simulink model "TOGGLER"  (R2022b)
settings: Solver=FixedStepDiscrete  StartTime=0  StopTime=duration  FixedStep=sample_time  RelTol=1e-3
values from neighbouring files (symbols this model uses):
  CTRL =     [TOGGLER_params.mat]
  CTRLSector =     [TOGGLER_params.mat]
  Greedy_Status = 1    [TOGGLER_params.mat]    (also in init_TOGGLER.m = logical(true))
  sample_time = 0.1    [TOGGLER_params.mat]
  WFC_1_Status = 1    [TOGGLER_params.mat]    (also in init_TOGGLER.m = logical(true))
  WFC_2_Status = 1    [TOGGLER_params.mat]    (also in init_TOGGLER.m = logical(true))
  WFC_3_Status = 1    [TOGGLER_params.mat]    (also in init_TOGGLER.m = logical(true))
undefined symbols (not defined in the file or in its folder): j
libraries: simulink x39, dspindex x14, dspstat3 x4, dspsigops x1
(part 2 of 2)

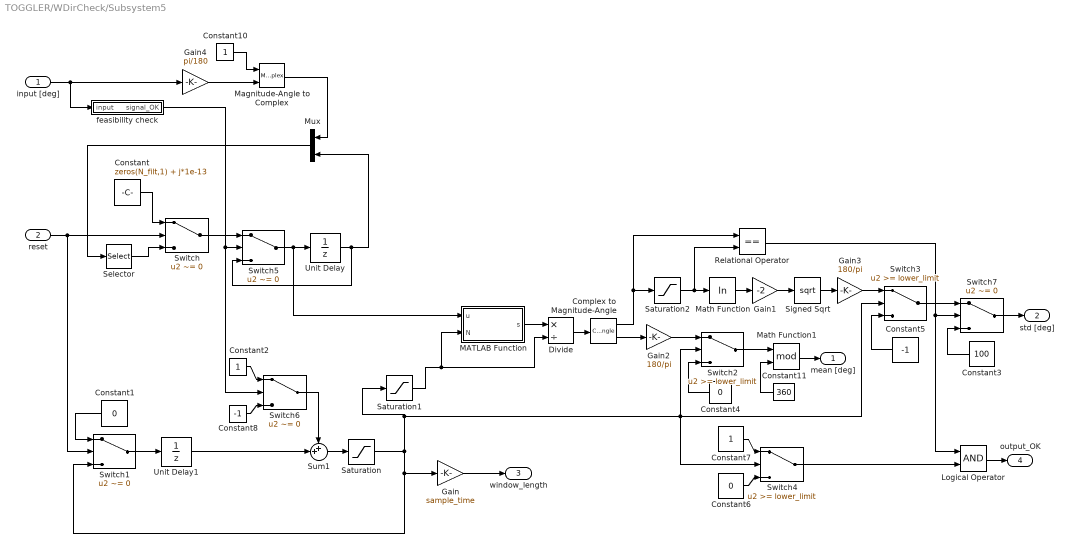
== system TOGGLER/WDirCheck/Subsystem5 ==
  input [deg] : Inport
  reset : Inport  Port=2
  Complex to Magnitude-Angle : ComplexToMagnitudeAngle
  Constant : Constant  Value=zeros(N_filt,1) + j*1e-13  SampleTime=sample_time
  Constant1 : Constant  Value=0  SampleTime=sample_time
  Constant10 : Constant  SampleTime=sample_time
  Constant11 : Constant  Value=360
  Constant2 : Constant  SampleTime=sample_time
  Constant3 : Constant  Value=100  SampleTime=sample_time
  Constant4 : Constant  Value=0  SampleTime=sample_time
  Constant5 : Constant  Value=-1  SampleTime=sample_time
  Constant6 : Constant  Value=0  OutDataTypeStr=boolean  SampleTime=sample_time
  Constant7 : Constant  OutDataTypeStr=boolean  SampleTime=sample_time
  Constant8 : Constant  Value=-1  SampleTime=sample_time
  Divide : Product  Inputs=*/
  Gain : Gain  Gain=sample_time
  Gain1 : Gain  Gain=-2
  Gain2 : Gain  Gain=180/pi
  Gain3 : Gain  Gain=180/pi
  Gain4 : Gain  Gain=pi/180
  Logical Operator : Logic  AllPortsSameDT=off  OutDataTypeStr=boolean
  MATLAB Function : MATLAB Function  TreatAsAtomicUnit=on
  Magnitude-Angle to Complex : MagnitudeAngleToComplex
  Math Function : Math  Operator=log  SignedPower=on
  Math Function1 : Math  Operator=mod  SignedPower=on
  Mux : Mux  Inputs=2
  Relational Operator : RelationalOperator  Operator===  OutDataTypeStr=boolean  RndMeth=Simplest  InputSameDT=off
  Saturation : Saturate  UpperLimit=N_filt  LowerLimit=0
  Saturation1 : Saturate  UpperLimit=N_filt  LowerLimit=lower_limit
  Saturation2 : Saturate  UpperLimit=1  LowerLimit=1e-7
  Selector : Selector  InputPortWidth=N_filt+1  IndexOptions=Index vector (dialog)  Indices=1:N_filt  OutputSizes=1
  Signed Sqrt : Sqrt
  Sum1 : Sum  Inputs=++|
  Switch{,1,5..6} (4 alike) : Switch  Criteria=u2 ~= 0  SaturateOnIntegerOverflow=off  InputSameDT=off
  Switch2 : Switch  Threshold=lower_limit  SaturateOnIntegerOverflow=off  InputSameDT=off
  Switch3 : Switch  Threshold=lower_limit  SaturateOnIntegerOverflow=off  InputSameDT=off
  Switch4 : Switch  Threshold=lower_limit  SaturateOnIntegerOverflow=off  InputSameDT=off
  Switch7 : Switch  Criteria=u2 ~= 0  Threshold=lower_limit  SaturateOnIntegerOverflow=off  InputSameDT=off
  Unit Delay : UnitDelay  InitialCondition=zeros(N_filt,1)  SampleTime=sample_time  HasFrameUpgradeWarning=on
  Unit Delay1 : UnitDelay  SampleTime=sample_time  HasFrameUpgradeWarning=on
  feasibility check : Subsystem
  mean [deg] : Outport
  std [deg] : Outport  Port=2
  window_length : Outport  Port=3
  output_OK : Outport  Port=4
  wires:
  Math Function1/1 -> mean [deg]/1
  Switch2/1 -> Math Function1/1
  Constant11/1 -> Math Function1/2
  Saturation2/1 -> Math Function/1, Relational Operator/2
  Gain3/1 -> Switch3/1
  Gain4/1 -> Magnitude-Angle to Complex/2
  input [deg]/1 -> Gain4/1, feasibility check/1(input)
  Gain2/1 -> Switch2/1
  Switch5/1 -> Unit Delay/1, MATLAB Function/1(u)
  Switch6/1 -> Sum1/1
  Constant7/1 -> Switch4/1
  Constant6/1 -> Switch4/3
  Constant1/1 -> Switch1/1
  Constant/1 -> Switch/1
  Selector/1 -> Switch/3
  Gain/1 -> window_length/1
  MATLAB Function/1(s) -> Divide/1
  Sum1/1 -> Saturation/1
  Signed Sqrt/1 -> Gain3/1
  Constant5/1 -> Switch3/3
  Switch1/1 -> Unit Delay1/1
  Switch3/1 -> Switch7/1
  Constant4/1 -> Switch2/3
  Unit Delay/1 -> Switch5/3, Mux/2
  Mux/1 -> Selector/1
  Saturation1/1 -> Divide/2, MATLAB Function/2(N)
  reset/1 -> Switch/2, Switch1/2
  Unit Delay1/1 -> Sum1/2
  Saturation/1 -> Gain/1, Switch1/3, Switch2/2, Switch4/2, Switch3/2, Saturation1/1
  feasibility check/1(signal_OK) -> Switch6/2, Switch5/2
  Switch/1 -> Switch5/1
  Constant2/1 -> Switch6/1
  Constant8/1 -> Switch6/3
  Magnitude-Angle to Complex/1 -> Mux/1
  Constant10/1 -> Magnitude-Angle to Complex/1
  Divide/1 -> Complex to Magnitude-Angle/1
  Complex to Magnitude-Angle/2 -> Gain2/1
  Complex to Magnitude-Angle/1 -> Saturation2/1, Relational Operator/1
  Math Function/1 -> Gain1/1
  Gain1/1 -> Signed Sqrt/1
  Logical Operator/1 -> output_OK/1
  Switch4/1 -> Logical Operator/2
  Relational Operator/1 -> Switch7/2, Logical Operator/1
  Constant3/1 -> Switch7/3
  Switch7/1 -> std [deg]/1

== system TOGGLER/Check Input/Subsystem5/Subsystem5 ==
  In1 : Inport
  Abs : Abs  SaturateOnIntegerOverflow=off
  Compare To Constant : simulink/Logic and Bit Operations/Compare To Constant  relop=<=  const=0.00001  OutDataTypeStr=boolean
  IsInf : RelationalOperator  Operator=isInf  OutDataTypeStr=boolean  RndMeth=Simplest  InputSameDT=off
  IsNaN : RelationalOperator  Operator=isNaN  OutDataTypeStr=boolean  RndMeth=Simplest  InputSameDT=off
  Logical Operator : Logic  Operator=OR  Inputs=3  AllPortsSameDT=off  OutDataTypeStr=boolean
  ErrorFlag : Outport  VectorParamsAs1DForOutWhenUnconnected=off
  wires:
  Abs/1 -> Compare To Constant/1
  Compare To Constant/1 -> Logical Operator/1
  Logical Operator/1 -> ErrorFlag/1
  IsInf/1 -> Logical Operator/3
  In1/1 -> IsInf/1, IsNaN/1, Abs/1
  IsNaN/1 -> Logical Operator/2

== system TOGGLER/Check Input/Subsystem6/Subsystem5 ==
  In1 : Inport
  Abs : Abs  SaturateOnIntegerOverflow=off
  Compare To Constant : simulink/Logic and Bit Operations/Compare To Constant  relop=<=  const=0.00001  OutDataTypeStr=boolean
  IsInf : RelationalOperator  Operator=isInf  OutDataTypeStr=boolean  RndMeth=Simplest  InputSameDT=off
  IsNaN : RelationalOperator  Operator=isNaN  OutDataTypeStr=boolean  RndMeth=Simplest  InputSameDT=off
  Logical Operator : Logic  Operator=OR  Inputs=3  AllPortsSameDT=off  OutDataTypeStr=boolean
  ErrorFlag : Outport  VectorParamsAs1DForOutWhenUnconnected=off
  wires:
  IsNaN/1 -> Logical Operator/2
  In1/1 -> Abs/1, IsNaN/1, IsInf/1
  IsInf/1 -> Logical Operator/3
  Logical Operator/1 -> ErrorFlag/1
  Compare To Constant/1 -> Logical Operator/1
  Abs/1 -> Compare To Constant/1

== system TOGGLER/CheckSectorsInflow/Atomic Subsystem/CheckRangeMisal ==
  VariableToCheck : Inport
  VarRange : Inport  Port=2  OutDataTypeStr=double
  IdxToCheck : Inport  Port=3
  Interval Test Dynamic : simulink/Logic and Bit Operations/Interval Test Dynamic  IntervalClosedRight=on  IntervalClosedLeft=on  OutDataTypeStr=boolean
  Scope : Scope  NumInputPorts=2
  Variable Selector3 : dspindex/Variable Selector  NumInputs=1  rowsOrCols=Rows  IdxMode=Variable  Elements=[1 3]  ZerOneIdxMode=One-based  errmode=Clip Index  FillMode=on  FillValues=0
  Zero : Constant  Value=0  OutDataTypeStr=Inherit: Inherit via back propagation
  Flag_InRange : Outport  VectorParamsAs1DForOutWhenUnconnected=off
  wires:
  IdxToCheck/1 -> Variable Selector3/2
  Interval Test Dynamic/1 -> Scope/1, Flag_InRange/1
  VarRange/1 -> Variable Selector3/1
  Variable Selector3/1 -> Interval Test Dynamic/1
  VariableToCheck/1 -> Scope/2, Interval Test Dynamic/2
  Zero/1 -> Interval Test Dynamic/3

== system TOGGLER/CheckSectorsInflow/Atomic Subsystem/CheckRangeNacelle ==
  VariableToCheck : Inport
  VarRange : Inport  Port=2  OutDataTypeStr=double
  IdxToCheck : Inport  Port=3
  Multiport Selector : dspindex/Multiport Selector  rowsOrCols=Columns  idxCellArray={ 1,2}  idxErrMode=Clip Index
  Scope : Scope  NumInputPorts=2
  Subsystem : Subsystem
  Variable Selector3 : dspindex/Variable Selector  NumInputs=1  rowsOrCols=Rows  IdxMode=Variable  Elements=[1 3]  ZerOneIdxMode=One-based  errmode=Clip Index  FillMode=on  FillValues=0
  Flag_InRange : Outport  VectorParamsAs1DForOutWhenUnconnected=off
  wires:
  IdxToCheck/1 -> Variable Selector3/2
  Multiport Selector/1 -> Subsystem/3(LowerBound)
  Subsystem/1(AngleInRange) -> Scope/1, Flag_InRange/1
  VarRange/1 -> Variable Selector3/1
  Variable Selector3/1 -> Multiport Selector/1
  Multiport Selector/2 -> Subsystem/1(UpperBound)
  VariableToCheck/1 -> Subsystem/2(Angle), Scope/2

== system TOGGLER/CheckSectorsInflow/Atomic Subsystem/CheckRangeWDir ==
  VariableToCheck : Inport
  VarRange : Inport  Port=2  OutDataTypeStr=double
  IdxToCheck : Inport  Port=3
  Multiport Selector : dspindex/Multiport Selector  rowsOrCols=Columns  idxCellArray={ 1,2}  idxErrMode=Clip Index
  Scope : Scope
  Subsystem : Subsystem
  Variable Selector3 : dspindex/Variable Selector  NumInputs=1  rowsOrCols=Rows  IdxMode=Variable  Elements=[1 3]  ZerOneIdxMode=One-based  errmode=Clip Index  FillMode=on  FillValues=0
  Flag_InRange : Outport  VectorParamsAs1DForOutWhenUnconnected=off
  wires:
  IdxToCheck/1 -> Variable Selector3/2
  Multiport Selector/1 -> Subsystem/3(LowerBound)
  VarRange/1 -> Variable Selector3/1
  Variable Selector3/1 -> Multiport Selector/1
  Multiport Selector/2 -> Subsystem/1(UpperBound)
  VariableToCheck/1 -> Subsystem/2(Angle)
  Subsystem/1(AngleInRange) -> Scope/1, Flag_InRange/1

== system TOGGLER/CheckSectorsInflow/Atomic Subsystem/CheckRangeWS ==
  VariableToCheck : Inport
  VarRange : Inport  Port=2  OutDataTypeStr=double
  IdxToCheck : Inport  Port=3
  Interval Test Dynamic : simulink/Logic and Bit Operations/Interval Test Dynamic  IntervalClosedRight=on  IntervalClosedLeft=on  OutDataTypeStr=boolean
  Multiport Selector : dspindex/Multiport Selector  rowsOrCols=Columns  idxCellArray={ 1,2}  idxErrMode=Clip Index
  Scope : Scope  NumInputPorts=2
  Variable Selector3 : dspindex/Variable Selector  NumInputs=1  rowsOrCols=Rows  IdxMode=Variable  Elements=[1 3]  ZerOneIdxMode=One-based  errmode=Clip Index  FillMode=on  FillValues=0
  Flag_InRange : Outport  VectorParamsAs1DForOutWhenUnconnected=off
  wires:
  IdxToCheck/1 -> Variable Selector3/2
  Multiport Selector/1 -> Interval Test Dynamic/3
  Interval Test Dynamic/1 -> Scope/2, Flag_InRange/1
  VarRange/1 -> Scope/1, Variable Selector3/1
  Variable Selector3/1 -> Multiport Selector/1
  Multiport Selector/2 -> Interval Test Dynamic/1
  VariableToCheck/1 -> Interval Test Dynamic/2

== system TOGGLER/CheckSectorsInflow/Atomic Subsystem1/CheckRangeMisal ==
  VariableToCheck : Inport
  VarRange : Inport  Port=2  OutDataTypeStr=double
  IdxToCheck : Inport  Port=3
  Interval Test Dynamic : simulink/Logic and Bit Operations/Interval Test Dynamic  IntervalClosedRight=on  IntervalClosedLeft=on  OutDataTypeStr=boolean
  Scope : Scope  NumInputPorts=2
  Variable Selector3 : dspindex/Variable Selector  NumInputs=1  rowsOrCols=Rows  IdxMode=Variable  Elements=[1 3]  ZerOneIdxMode=One-based  errmode=Clip Index  FillMode=on  FillValues=0
  Zero : Constant  Value=0  OutDataTypeStr=Inherit: Inherit via back propagation
  Flag_InRange : Outport  VectorParamsAs1DForOutWhenUnconnected=off
  wires:
  Zero/1 -> Interval Test Dynamic/3
  VariableToCheck/1 -> Interval Test Dynamic/2, Scope/2
  Variable Selector3/1 -> Interval Test Dynamic/1
  VarRange/1 -> Variable Selector3/1
  Interval Test Dynamic/1 -> Flag_InRange/1, Scope/1
  IdxToCheck/1 -> Variable Selector3/2

== system TOGGLER/CheckSectorsInflow/Atomic Subsystem1/CheckRangeNacelle ==
  VariableToCheck : Inport
  VarRange : Inport  Port=2  OutDataTypeStr=double
  IdxToCheck : Inport  Port=3
  Multiport Selector : dspindex/Multiport Selector  rowsOrCols=Columns  idxCellArray={ 1,2}  idxErrMode=Clip Index
  Scope : Scope  NumInputPorts=2
  Subsystem : Subsystem
  Variable Selector3 : dspindex/Variable Selector  NumInputs=1  rowsOrCols=Rows  IdxMode=Variable  Elements=[1 3]  ZerOneIdxMode=One-based  errmode=Clip Index  FillMode=on  FillValues=0
  Flag_InRange : Outport  VectorParamsAs1DForOutWhenUnconnected=off
  wires:
  VariableToCheck/1 -> Subsystem/2(Angle), Scope/2
  Variable Selector3/1 -> Multiport Selector/1
  VarRange/1 -> Variable Selector3/1
  Subsystem/1(AngleInRange) -> Scope/1, Flag_InRange/1
  IdxToCheck/1 -> Variable Selector3/2
  Multiport Selector/1 -> Subsystem/3(LowerBound)
  Multiport Selector/2 -> Subsystem/1(UpperBound)

== system TOGGLER/CheckSectorsInflow/Atomic Subsystem1/CheckRangeWDir ==
  VariableToCheck : Inport
  VarRange : Inport  Port=2  OutDataTypeStr=double
  IdxToCheck : Inport  Port=3
  Multiport Selector : dspindex/Multiport Selector  rowsOrCols=Columns  idxCellArray={ 1,2}  idxErrMode=Clip Index
  Scope : Scope
  Scope1 : Scope  NumInputPorts=3
  Subsystem : Subsystem
  Variable Selector3 : dspindex/Variable Selector  NumInputs=1  rowsOrCols=Rows  IdxMode=Variable  Elements=[1 3]  ZerOneIdxMode=One-based  errmode=Clip Index  FillMode=on  FillValues=0
  Flag_InRange : Outport  VectorParamsAs1DForOutWhenUnconnected=off
  wires:
  VariableToCheck/1 -> Scope1/3, Subsystem/2(Angle)
  Multiport Selector/2 -> Scope1/2, Subsystem/1(UpperBound)
  Variable Selector3/1 -> Multiport Selector/1
  VarRange/1 -> Variable Selector3/1
  Subsystem/1(AngleInRange) -> Flag_InRange/1, Scope/1
  Multiport Selector/1 -> Scope1/1, Subsystem/3(LowerBound)
  IdxToCheck/1 -> Variable Selector3/2

== system TOGGLER/CheckSectorsInflow/Atomic Subsystem1/CheckRangeWS ==
  VariableToCheck : Inport
  VarRange : Inport  Port=2  OutDataTypeStr=double
  IdxToCheck : Inport  Port=3
  Interval Test Dynamic : simulink/Logic and Bit Operations/Interval Test Dynamic  IntervalClosedRight=on  IntervalClosedLeft=on  OutDataTypeStr=boolean
  Multiport Selector : dspindex/Multiport Selector  rowsOrCols=Columns  idxCellArray={ 1,2}  idxErrMode=Clip Index
  Scope : Scope  NumInputPorts=2
  Variable Selector3 : dspindex/Variable Selector  NumInputs=1  rowsOrCols=Rows  IdxMode=Variable  Elements=[1 3]  ZerOneIdxMode=One-based  errmode=Clip Index  FillMode=on  FillValues=0
  Flag_InRange : Outport  VectorParamsAs1DForOutWhenUnconnected=off
  wires:
  VariableToCheck/1 -> Interval Test Dynamic/2
  Multiport Selector/2 -> Interval Test Dynamic/1
  Variable Selector3/1 -> Multiport Selector/1
  VarRange/1 -> Variable Selector3/1, Scope/1
  Interval Test Dynamic/1 -> Flag_InRange/1, Scope/2
  Multiport Selector/1 -> Interval Test Dynamic/3
  IdxToCheck/1 -> Variable Selector3/2

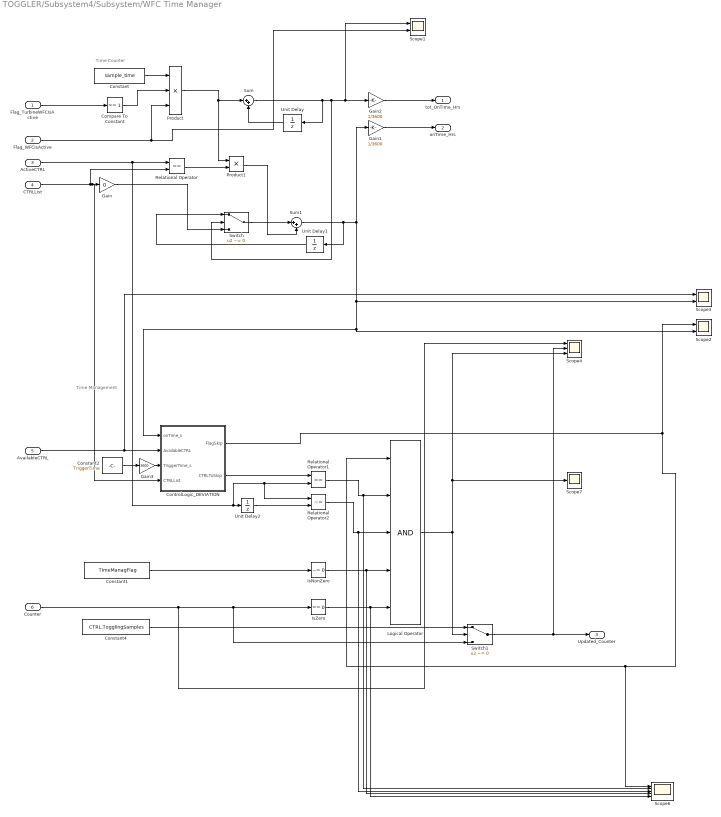
== system TOGGLER/Subsystem4/Subsystem/WFC Time Manager ==
  note: Time Counter
  note: Time Management
  Flag_TurbineWFCIsActive : Inport
  Flag_WFCIsActive : Inport  Port=2
  ActiveCTRL : Inport  Port=3
  CTRLList : Inport  Port=4
  AvailableCTRL : Inport  Port=5
  Counter : Inport  Port=6
  Compare To Constant : simulink/Logic and Bit Operations/Compare To Constant  relop===  const=1  OutDataTypeStr=boolean
  Constant : Constant  Value=sample_time
  Constant1 : Constant  Value=TimeManagFlag
  Constant2 : Constant  Value=TriggerTime
  Constant4 : Constant  Value=CTRL.TogglingSamples
  ControlLogic_DEVIATION : Subsystem
  Gain : Gain  Gain=0
  Gain1 : Gain  Gain=1/3600
  Gain2 : Gain  Gain=1/3600
  Gain3 : Gain  Gain=3600
  IsNonZero : simulink/Logic and Bit Operations/Compare To Zero  relop=~=  OutDataTypeStr=boolean
  IsZero : simulink/Logic and Bit Operations/Compare To Zero  relop===  OutDataTypeStr=boolean
  Logical Operator : Logic  Inputs=5  AllPortsSameDT=off  OutDataTypeStr=boolean
  Product : Product  Inputs=3
  Product1 : Product
  Relational Operator : RelationalOperator  Operator===  OutDataTypeStr=boolean  RndMeth=Simplest  InputSameDT=off
  Relational Operator1 : RelationalOperator  Operator===  OutDataTypeStr=boolean  RndMeth=Simplest  InputSameDT=off
  Relational Operator2 : RelationalOperator  Operator=~=  OutDataTypeStr=boolean  RndMeth=Simplest  InputSameDT=off
  Scope1 : Scope  NumInputPorts=2
  Scope2 : Scope  NumInputPorts=2
  Scope3 : Scope  NumInputPorts=2
  Scope4 : Scope  NumInputPorts=3
  Scope6 : Scope  NumInputPorts=5
  Scope7 : Scope
  Sum : Sum  Inputs=|++
  Sum1 : Sum  Inputs=|++
  Switch : Switch  Criteria=u2 ~= 0  SaturateOnIntegerOverflow=off  InputSameDT=off
  Switch1 : Switch  Criteria=u2 ~= 0  SaturateOnIntegerOverflow=off  InputSameDT=off
  Unit Delay : UnitDelay  SampleTime=-1  HasFrameUpgradeWarning=on
  Unit Delay1 : UnitDelay  SampleTime=-1  HasFrameUpgradeWarning=on
  Unit Delay2 : UnitDelay  SampleTime=-1  HasFrameUpgradeWarning=on
  tot_OnTime_Hrs : Outport  VectorParamsAs1DForOutWhenUnconnected=off
  onTime_Hrs : Outport  Port=2  VectorParamsAs1DForOutWhenUnconnected=off
  Updated_Counter : Outport  Port=3  VectorParamsAs1DForOutWhenUnconnected=off
  wires:
  Flag_WFCIsActive/1 -> Product/3, Scope1/2
  Constant/1 -> Product/1
  CTRLList/1 -> ControlLogic_DEVIATION/4(CTRLList), Gain/1, Relational Operator/2
  Gain/1 -> Switch/3
  Switch/1 -> Sum1/1
  Unit Delay/1 -> Sum/2
  Sum/1 -> Unit Delay/1, Switch/2, Scope1/1, Gain2/1
  Product/1 -> Product1/1, Sum/1
  ActiveCTRL/1 -> Relational Operator/1, Relational Operator2/1, Relational Operator1/2, Unit Delay2/1
  Sum1/1 -> Scope2/2, ControlLogic_DEVIATION/1(onTime_s), Scope3/2, Gain1/1, Unit Delay1/1
  Unit Delay1/1 -> Switch/1
  Relational Operator/1 -> Product1/2
  Product1/1 -> Sum1/2
  Gain1/1 -> onTime_Hrs/1
  Gain2/1 -> tot_OnTime_Hrs/1
  Constant1/1 -> IsNonZero/1
  Constant2/1 -> Gain3/1
  Unit Delay2/1 -> Relational Operator2/2
  ControlLogic_DEVIATION/1(FlagSkip) -> Scope2/1, Scope6/1, Logical Operator/1
  AvailableCTRL/1 -> Scope3/1, ControlLogic_DEVIATION/2(AvailableCTRL)
  Gain3/1 -> ControlLogic_DEVIATION/3(TriggerTime_s)
  Relational Operator1/1 -> Scope6/2, Logical Operator/2
  Relational Operator2/1 -> Logical Operator/3, Scope6/3
  IsNonZero/1 -> Logical Operator/4, Scope6/4
  Counter/1 -> Switch1/3, IsZero/1, Scope4/1
  IsZero/1 -> Logical Operator/5, Scope6/5
  Logical Operator/1 -> Scope4/3, Scope7/1, Switch1/2
  Constant4/1 -> Switch1/1
  Switch1/1 -> Scope4/2, Updated_Counter/1
  ControlLogic_DEVIATION/2(CTRLToSkip) -> Relational Operator1/1
  Flag_TurbineWFCIsActive/1 -> Compare To Constant/1
  Compare To Constant/1 -> Product/2

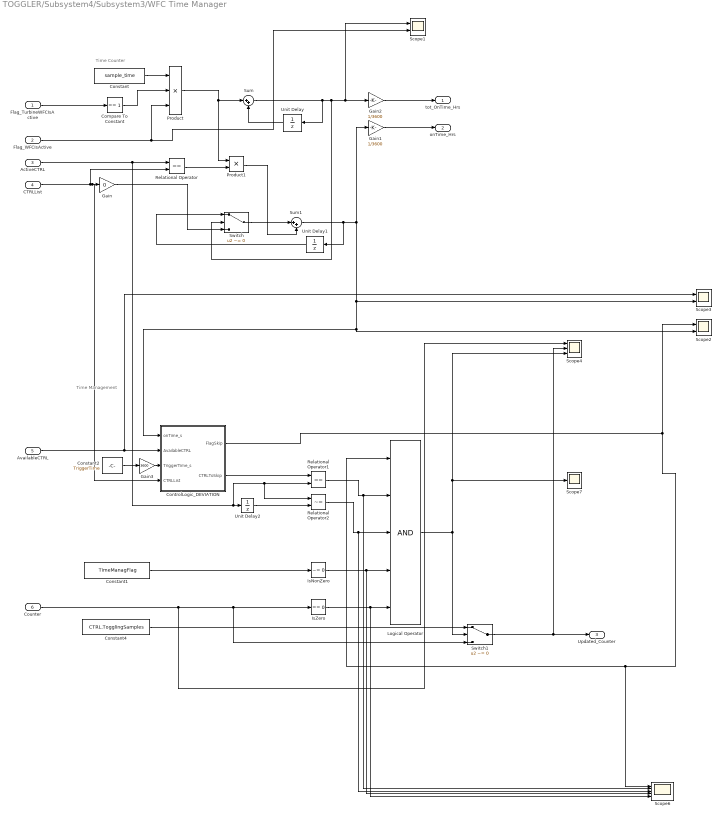
== system TOGGLER/Subsystem4/Subsystem3/WFC Time Manager ==
  note: Time Management
  note: Time Counter
  Flag_TurbineWFCIsActive : Inport
  Flag_WFCIsActive : Inport  Port=2
  ActiveCTRL : Inport  Port=3
  CTRLList : Inport  Port=4
  AvailableCTRL : Inport  Port=5
  Counter : Inport  Port=6
  Compare To Constant : simulink/Logic and Bit Operations/Compare To Constant  relop===  const=1  OutDataTypeStr=boolean
  Constant : Constant  Value=sample_time
  Constant1 : Constant  Value=TimeManagFlag
  Constant2 : Constant  Value=TriggerTime
  Constant4 : Constant  Value=CTRL.TogglingSamples
  ControlLogic_DEVIATION : Subsystem
  Gain : Gain  Gain=0
  Gain1 : Gain  Gain=1/3600
  Gain2 : Gain  Gain=1/3600
  Gain3 : Gain  Gain=3600
  IsNonZero : simulink/Logic and Bit Operations/Compare To Zero  relop=~=  OutDataTypeStr=boolean
  IsZero : simulink/Logic and Bit Operations/Compare To Zero  relop===  OutDataTypeStr=boolean
  Logical Operator : Logic  Inputs=5  AllPortsSameDT=off  OutDataTypeStr=boolean
  Product : Product  Inputs=3
  Product1 : Product
  Relational Operator : RelationalOperator  Operator===  OutDataTypeStr=boolean  RndMeth=Simplest  InputSameDT=off
  Relational Operator1 : RelationalOperator  Operator===  OutDataTypeStr=boolean  RndMeth=Simplest  InputSameDT=off
  Relational Operator2 : RelationalOperator  Operator=~=  OutDataTypeStr=boolean  RndMeth=Simplest  InputSameDT=off
  Scope1 : Scope  NumInputPorts=2
  Scope2 : Scope  NumInputPorts=2
  Scope3 : Scope  NumInputPorts=2
  Scope4 : Scope  NumInputPorts=3
  Scope6 : Scope  NumInputPorts=5
  Scope7 : Scope
  Sum : Sum  Inputs=|++
  Sum1 : Sum  Inputs=|++
  Switch : Switch  Criteria=u2 ~= 0  SaturateOnIntegerOverflow=off  InputSameDT=off
  Switch1 : Switch  Criteria=u2 ~= 0  SaturateOnIntegerOverflow=off  InputSameDT=off
  Unit Delay : UnitDelay  SampleTime=-1  HasFrameUpgradeWarning=on
  Unit Delay1 : UnitDelay  SampleTime=-1  HasFrameUpgradeWarning=on
  Unit Delay2 : UnitDelay  SampleTime=-1  HasFrameUpgradeWarning=on
  tot_OnTime_Hrs : Outport  VectorParamsAs1DForOutWhenUnconnected=off
  onTime_Hrs : Outport  Port=2  VectorParamsAs1DForOutWhenUnconnected=off
  Updated_Counter : Outport  Port=3  VectorParamsAs1DForOutWhenUnconnected=off
  wires:
  Compare To Constant/1 -> Product/2
  Flag_TurbineWFCIsActive/1 -> Compare To Constant/1
  ControlLogic_DEVIATION/2(CTRLToSkip) -> Relational Operator1/1
  Switch1/1 -> Updated_Counter/1, Scope4/2
  Constant4/1 -> Switch1/1
  Logical Operator/1 -> Switch1/2, Scope7/1, Scope4/3
  IsZero/1 -> Scope6/5, Logical Operator/5
  Counter/1 -> Scope4/1, IsZero/1, Switch1/3
  IsNonZero/1 -> Scope6/4, Logical Operator/4
  Relational Operator2/1 -> Scope6/3, Logical Operator/3
  Relational Operator1/1 -> Logical Operator/2, Scope6/2
  Gain3/1 -> ControlLogic_DEVIATION/3(TriggerTime_s)
  AvailableCTRL/1 -> ControlLogic_DEVIATION/2(AvailableCTRL), Scope3/1
  ControlLogic_DEVIATION/1(FlagSkip) -> Logical Operator/1, Scope6/1, Scope2/1
  Unit Delay2/1 -> Relational Operator2/2
  Constant2/1 -> Gain3/1
  Constant1/1 -> IsNonZero/1
  Gain2/1 -> tot_OnTime_Hrs/1
  Gain1/1 -> onTime_Hrs/1
  Product1/1 -> Sum1/2
  Relational Operator/1 -> Product1/2
  Unit Delay1/1 -> Switch/1
  Sum1/1 -> Unit Delay1/1, Gain1/1, Scope3/2, ControlLogic_DEVIATION/1(onTime_s), Scope2/2
  ActiveCTRL/1 -> Unit Delay2/1, Relational Operator1/2, Relational Operator2/1, Relational Operator/1
  Product/1 -> Sum/1, Product1/1
  Sum/1 -> Gain2/1, Scope1/1, Switch/2, Unit Delay/1
  Unit Delay/1 -> Sum/2
  Switch/1 -> Sum1/1
  Gain/1 -> Switch/3
  CTRLList/1 -> Relational Operator/2, Gain/1, ControlLogic_DEVIATION/4(CTRLList)
  Constant/1 -> Product/1
  Flag_WFCIsActive/1 -> Scope1/2, Product/3

== system TOGGLER/WDirCheck/Subsystem5/feasibility check ==
  input : Inport
  Abs : Abs  SaturateOnIntegerOverflow=off
  Compare To Constant : simulink/Logic and Bit Operations/Compare To Constant  relop=<  const=inf  OutDataTypeStr=boolean
  Compare To Constant1 : simulink/Logic and Bit Operations/Compare To Constant  relop=>  const=-inf  OutDataTypeStr=boolean
  Compare To Constant2 : simulink/Logic and Bit Operations/Compare To Constant  relop=<=  const=420  OutDataTypeStr=boolean
  Logical Operator : Logic  Inputs=4  AllPortsSameDT=off  OutDataTypeStr=boolean
  Relational Operator : RelationalOperator  Operator===  OutDataTypeStr=boolean  RndMeth=Simplest  InputSameDT=off
  Sum : Sum  Inputs=-+|
  Unit Delay : UnitDelay  SampleTime=sample_time  HasFrameUpgradeWarning=on
  signal_OK : Outport
  wires:
  Compare To Constant2/1 -> Logical Operator/1
  Abs/1 -> Compare To Constant2/1
  Sum/1 -> Abs/1
  Unit Delay/1 -> Sum/1
  input/1 -> Compare To Constant1/1, Compare To Constant/1, Relational Operator/2, Relational Operator/1, Unit Delay/1, Sum/2
  Compare To Constant/1 -> Logical Operator/3
  Logical Operator/1 -> signal_OK/1
  Relational Operator/1 -> Logical Operator/2
  Compare To Constant1/1 -> Logical Operator/4

== system TOGGLER/CheckSectorsInflow/Atomic Subsystem/CheckRangeNacelle/Subsystem ==
  UpperBound : Inport
  Angle : Inport  Port=2
  LowerBound : Inport  Port=3
  Logical Operator : Logic  AllPortsSameDT=off  OutDataTypeStr=boolean
  Logical Operator1 : Logic  Operator=OR  AllPortsSameDT=off  OutDataTypeStr=boolean
  Relational Operator : RelationalOperator  OutDataTypeStr=boolean  RndMeth=Simplest  InputSameDT=off
  Relational Operator1 : RelationalOperator  OutDataTypeStr=boolean  RndMeth=Simplest  InputSameDT=off
  Relational Operator2 : RelationalOperator  Operator=<=  OutDataTypeStr=boolean  RndMeth=Simplest  InputSameDT=off
  Subtract : Sum  Inputs=+-
  Switch : Switch  Criteria=u2 ~= 0  SaturateOnIntegerOverflow=off  InputSameDT=off
  Zero : Constant  Value=0  OutDataTypeStr=Inherit: Inherit via back propagation
  AngleInRange : Outport  VectorParamsAs1DForOutWhenUnconnected=off
  wires:
  Angle/1 -> Relational Operator1/1, Relational Operator2/1
  Subtract/1 -> Relational Operator/1
  Switch/1 -> AngleInRange/1
  Relational Operator2/1 -> Logical Operator1/2, Logical Operator/2
  Relational Operator1/1 -> Logical Operator1/1, Logical Operator/1
  LowerBound/1 -> Subtract/2, Relational Operator1/2
  Zero/1 -> Relational Operator/2
  UpperBound/1 -> Relational Operator2/2, Subtract/1
  Logical Operator1/1 -> Switch/3
  Relational Operator/1 -> Switch/2
  Logical Operator/1 -> Switch/1

== system TOGGLER/CheckSectorsInflow/Atomic Subsystem/CheckRangeWDir/Subsystem ==
  UpperBound : Inport
  Angle : Inport  Port=2
  LowerBound : Inport  Port=3
  Logical Operator : Logic  AllPortsSameDT=off  OutDataTypeStr=boolean
  Logical Operator1 : Logic  Operator=OR  AllPortsSameDT=off  OutDataTypeStr=boolean
  Relational Operator : RelationalOperator  OutDataTypeStr=boolean  RndMeth=Simplest  InputSameDT=off
  Relational Operator1 : RelationalOperator  OutDataTypeStr=boolean  RndMeth=Simplest  InputSameDT=off
  Relational Operator2 : RelationalOperator  Operator=<=  OutDataTypeStr=boolean  RndMeth=Simplest  InputSameDT=off
  Subtract : Sum  Inputs=+-
  Switch : Switch  Criteria=u2 ~= 0  SaturateOnIntegerOverflow=off  InputSameDT=off
  Zero : Constant  Value=0  OutDataTypeStr=Inherit: Inherit via back propagation
  AngleInRange : Outport  VectorParamsAs1DForOutWhenUnconnected=off
  wires:
  Angle/1 -> Relational Operator1/1, Relational Operator2/1
  Subtract/1 -> Relational Operator/1
  Switch/1 -> AngleInRange/1
  Relational Operator2/1 -> Logical Operator1/2, Logical Operator/2
  Relational Operator1/1 -> Logical Operator1/1, Logical Operator/1
  LowerBound/1 -> Subtract/2, Relational Operator1/2
  Zero/1 -> Relational Operator/2
  UpperBound/1 -> Relational Operator2/2, Subtract/1
  Logical Operator1/1 -> Switch/3
  Relational Operator/1 -> Switch/2
  Logical Operator/1 -> Switch/1

== system TOGGLER/CheckSectorsInflow/Atomic Subsystem1/CheckRangeNacelle/Subsystem ==
  UpperBound : Inport
  Angle : Inport  Port=2
  LowerBound : Inport  Port=3
  Logical Operator : Logic  AllPortsSameDT=off  OutDataTypeStr=boolean
  Logical Operator1 : Logic  Operator=OR  AllPortsSameDT=off  OutDataTypeStr=boolean
  Relational Operator : RelationalOperator  OutDataTypeStr=boolean  RndMeth=Simplest  InputSameDT=off
  Relational Operator1 : RelationalOperator  OutDataTypeStr=boolean  RndMeth=Simplest  InputSameDT=off
  Relational Operator2 : RelationalOperator  Operator=<=  OutDataTypeStr=boolean  RndMeth=Simplest  InputSameDT=off
  Subtract : Sum  Inputs=+-
  Switch : Switch  Criteria=u2 ~= 0  SaturateOnIntegerOverflow=off  InputSameDT=off
  Zero : Constant  Value=0  OutDataTypeStr=Inherit: Inherit via back propagation
  AngleInRange : Outport  VectorParamsAs1DForOutWhenUnconnected=off
  wires:
  Angle/1 -> Relational Operator1/1, Relational Operator2/1
  Subtract/1 -> Relational Operator/1
  Switch/1 -> AngleInRange/1
  Relational Operator2/1 -> Logical Operator1/2, Logical Operator/2
  Relational Operator1/1 -> Logical Operator1/1, Logical Operator/1
  LowerBound/1 -> Subtract/2, Relational Operator1/2
  Zero/1 -> Relational Operator/2
  UpperBound/1 -> Relational Operator2/2, Subtract/1
  Logical Operator1/1 -> Switch/3
  Relational Operator/1 -> Switch/2
  Logical Operator/1 -> Switch/1

== system TOGGLER/CheckSectorsInflow/Atomic Subsystem1/CheckRangeWDir/Subsystem ==
  UpperBound : Inport
  Angle : Inport  Port=2
  LowerBound : Inport  Port=3
  Logical Operator : Logic  AllPortsSameDT=off  OutDataTypeStr=boolean
  Logical Operator1 : Logic  Operator=OR  AllPortsSameDT=off  OutDataTypeStr=boolean
  Relational Operator : RelationalOperator  OutDataTypeStr=boolean  RndMeth=Simplest  InputSameDT=off
  Relational Operator1 : RelationalOperator  OutDataTypeStr=boolean  RndMeth=Simplest  InputSameDT=off
  Relational Operator2 : RelationalOperator  Operator=<=  OutDataTypeStr=boolean  RndMeth=Simplest  InputSameDT=off
  Subtract : Sum  Inputs=+-
  Switch : Switch  Criteria=u2 ~= 0  SaturateOnIntegerOverflow=off  InputSameDT=off
  Zero : Constant  Value=0  OutDataTypeStr=Inherit: Inherit via back propagation
  AngleInRange : Outport  VectorParamsAs1DForOutWhenUnconnected=off
  wires:
  Angle/1 -> Relational Operator1/1, Relational Operator2/1
  Subtract/1 -> Relational Operator/1
  Switch/1 -> AngleInRange/1
  Relational Operator2/1 -> Logical Operator1/2, Logical Operator/2
  Relational Operator1/1 -> Logical Operator1/1, Logical Operator/1
  LowerBound/1 -> Subtract/2, Relational Operator1/2
  Zero/1 -> Relational Operator/2
  UpperBound/1 -> Relational Operator2/2, Subtract/1
  Logical Operator1/1 -> Switch/3
  Relational Operator/1 -> Switch/2
  Logical Operator/1 -> Switch/1

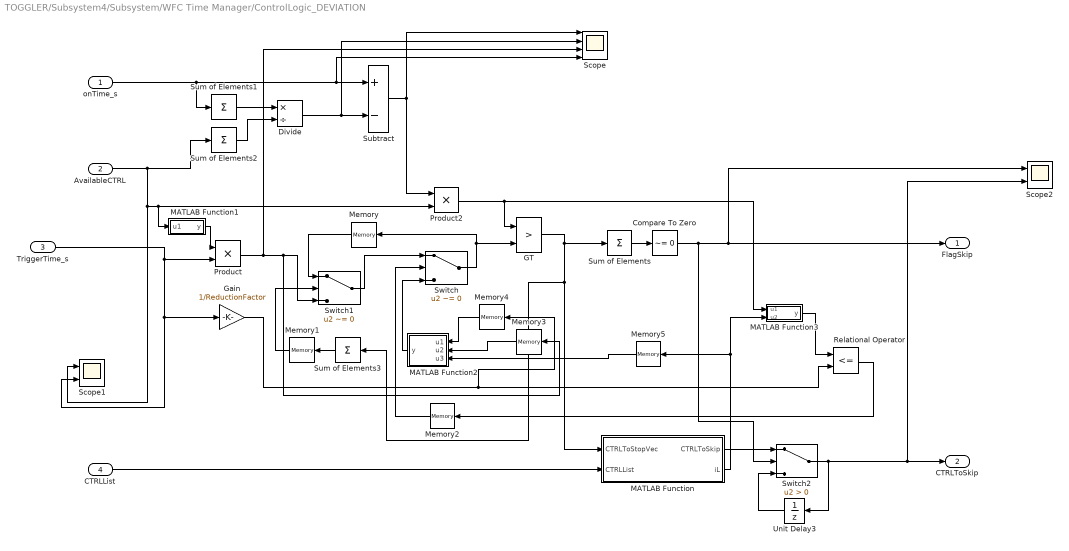
== system TOGGLER/Subsystem4/Subsystem/WFC Time Manager/ControlLogic_DEVIATION ==
  onTime_s : Inport
  AvailableCTRL : Inport  Port=2
  TriggerTime_s : Inport  Port=3
  CTRLList : Inport  Port=4
  Compare To Zero : simulink/Logic and Bit Operations/Compare To Zero  relop=~=  OutDataTypeStr=boolean
  Divide : Product  Inputs=*/
  GT : RelationalOperator  Operator=>  OutDataTypeStr=boolean  RndMeth=Simplest  InputSameDT=off
  Gain : Gain  Gain=1/ReductionFactor
  MATLAB Function : MATLAB Function  TreatAsAtomicUnit=on
  MATLAB Function1 : MATLAB Function  TreatAsAtomicUnit=on
  MATLAB Function2 : MATLAB Function  TreatAsAtomicUnit=on
  MATLAB Function3 : MATLAB Function  TreatAsAtomicUnit=on
  Memory{,1,3..5} (5 alike) : Memory
  Memory2 : Memory  InitialCondition=1
  Product : Product
  Product2 : Product
  Relational Operator : RelationalOperator  Operator=<=  OutDataTypeStr=boolean  RndMeth=Simplest  InputSameDT=off
  Scope : Scope  NumInputPorts=4
  Scope1 : Scope  NumInputPorts=2
  Scope2 : Scope  NumInputPorts=2
  Subtract : Sum  Inputs=+-
  Sum of Elements{,1..3} (4 alike) : Sum  Inputs=+
  Switch : Switch  Criteria=u2 ~= 0  SaturateOnIntegerOverflow=off  InputSameDT=off
  Switch1 : Switch  Criteria=u2 ~= 0  SaturateOnIntegerOverflow=off  InputSameDT=off
  Switch2 : Switch  Criteria=u2 > Threshold  SaturateOnIntegerOverflow=off  InputSameDT=off
  Unit Delay3 : UnitDelay  SampleTime=-1  HasFrameUpgradeWarning=on
  FlagSkip : Outport  VectorParamsAs1DForOutWhenUnconnected=off
  CTRLToSkip : Outport  Port=2  VectorParamsAs1DForOutWhenUnconnected=off
  wires:
  Divide/1 -> Subtract/2, Scope/2
  AvailableCTRL/1 -> Sum of Elements2/1, Product2/2, MATLAB Function1/1(u1), Scope1/1
  Subtract/1 -> Product2/1, Scope/1
  Product2/1 -> MATLAB Function3/1(u1), GT/1
  TriggerTime_s/1 -> Product/2, Gain/1, Scope1/2
  Sum of Elements/1 -> Compare To Zero/1
  onTime_s/1 -> Sum of Elements1/1, Subtract/1, Scope/4
  Sum of Elements1/1 -> Divide/1
  Sum of Elements2/1 -> Divide/2
  Switch2/1 -> Scope2/2, CTRLToSkip/1, Unit Delay3/1
  MATLAB Function/1(CTRLToSkip) -> Switch2/1
  Compare To Zero/1 -> FlagSkip/1, Scope2/1, Switch2/2
  Unit Delay3/1 -> Switch2/3
  CTRLList/1 -> MATLAB Function/2(CTRLList)
  MATLAB Function/2(iL) -> MATLAB Function3/2(u2), Memory5/1
  MATLAB Function3/1(y) -> Relational Operator/1
  MATLAB Function1/1(y) -> Product/1
  Product/1 -> Memory3/1, Switch1/3, Scope/3
  Gain/1 -> Memory4/1, Relational Operator/2
  Memory2/1 -> Switch/2
  Switch/1 -> GT/2, Memory/1
  MATLAB Function2/1(y) -> Switch/3
  Memory/1 -> Switch1/1
  Switch1/1 -> Switch/1
  Sum of Elements3/1 -> Memory1/1
  Memory1/1 -> Switch1/2
  Relational Operator/1 -> Memory2/1
  Memory3/1 -> MATLAB Function2/2(u2)
  Memory4/1 -> MATLAB Function2/1(u1)
  Memory5/1 -> MATLAB Function2/3(u3)
  GT/1 -> Sum of Elements3/1, MATLAB Function/1(CTRLToStopVec), Sum of Elements/1

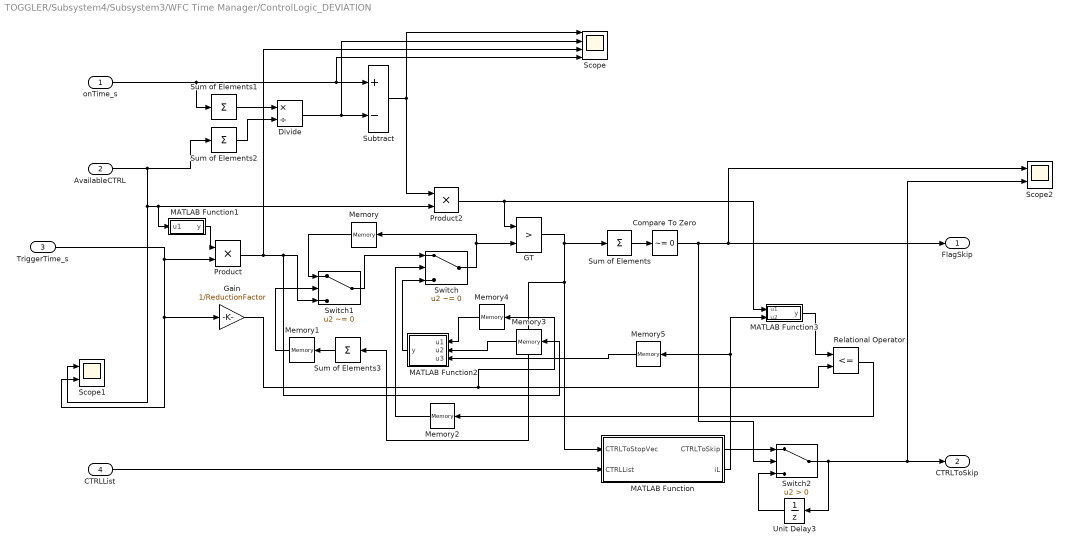
== system TOGGLER/Subsystem4/Subsystem3/WFC Time Manager/ControlLogic_DEVIATION ==
  onTime_s : Inport
  AvailableCTRL : Inport  Port=2
  TriggerTime_s : Inport  Port=3
  CTRLList : Inport  Port=4
  Compare To Zero : simulink/Logic and Bit Operations/Compare To Zero  relop=~=  OutDataTypeStr=boolean
  Divide : Product  Inputs=*/
  GT : RelationalOperator  Operator=>  OutDataTypeStr=boolean  RndMeth=Simplest  InputSameDT=off
  Gain : Gain  Gain=1/ReductionFactor
  MATLAB Function : MATLAB Function  TreatAsAtomicUnit=on
  MATLAB Function1 : MATLAB Function  TreatAsAtomicUnit=on
  MATLAB Function2 : MATLAB Function  TreatAsAtomicUnit=on
  MATLAB Function3 : MATLAB Function  TreatAsAtomicUnit=on
  Memory{,1,3..5} (5 alike) : Memory
  Memory2 : Memory  InitialCondition=1
  Product : Product
  Product2 : Product
  Relational Operator : RelationalOperator  Operator=<=  OutDataTypeStr=boolean  RndMeth=Simplest  InputSameDT=off
  Scope : Scope  NumInputPorts=4
  Scope1 : Scope  NumInputPorts=2
  Scope2 : Scope  NumInputPorts=2
  Subtract : Sum  Inputs=+-
  Sum of Elements{,1..3} (4 alike) : Sum  Inputs=+
  Switch : Switch  Criteria=u2 ~= 0  SaturateOnIntegerOverflow=off  InputSameDT=off
  Switch1 : Switch  Criteria=u2 ~= 0  SaturateOnIntegerOverflow=off  InputSameDT=off
  Switch2 : Switch  Criteria=u2 > Threshold  SaturateOnIntegerOverflow=off  InputSameDT=off
  Unit Delay3 : UnitDelay  SampleTime=-1  HasFrameUpgradeWarning=on
  FlagSkip : Outport  VectorParamsAs1DForOutWhenUnconnected=off
  CTRLToSkip : Outport  Port=2  VectorParamsAs1DForOutWhenUnconnected=off
  wires:
  GT/1 -> Sum of Elements/1, MATLAB Function/1(CTRLToStopVec), Sum of Elements3/1
  Memory5/1 -> MATLAB Function2/3(u3)
  Memory4/1 -> MATLAB Function2/1(u1)
  Memory3/1 -> MATLAB Function2/2(u2)
  Relational Operator/1 -> Memory2/1
  Memory1/1 -> Switch1/2
  Sum of Elements3/1 -> Memory1/1
  Switch1/1 -> Switch/1
  Memory/1 -> Switch1/1
  MATLAB Function2/1(y) -> Switch/3
  Switch/1 -> Memory/1, GT/2
  Memory2/1 -> Switch/2
  Gain/1 -> Relational Operator/2, Memory4/1
  Product/1 -> Scope/3, Switch1/3, Memory3/1
  MATLAB Function1/1(y) -> Product/1
  MATLAB Function3/1(y) -> Relational Operator/1
  MATLAB Function/2(iL) -> Memory5/1, MATLAB Function3/2(u2)
  CTRLList/1 -> MATLAB Function/2(CTRLList)
  Unit Delay3/1 -> Switch2/3
  Compare To Zero/1 -> Switch2/2, Scope2/1, FlagSkip/1
  MATLAB Function/1(CTRLToSkip) -> Switch2/1
  Switch2/1 -> Unit Delay3/1, CTRLToSkip/1, Scope2/2
  Sum of Elements2/1 -> Divide/2
  Sum of Elements1/1 -> Divide/1
  onTime_s/1 -> Scope/4, Subtract/1, Sum of Elements1/1
  Sum of Elements/1 -> Compare To Zero/1
  TriggerTime_s/1 -> Scope1/2, Gain/1, Product/2
  Product2/1 -> GT/1, MATLAB Function3/1(u1)
  Subtract/1 -> Scope/1, Product2/1
  AvailableCTRL/1 -> Scope1/1, MATLAB Function1/1(u1), Product2/2, Sum of Elements2/1
  Divide/1 -> Scope/2, Subtract/2

== matlab function TOGGLER/Subsystem4/Subsystem3/WFC Time Manager/ControlLogic_DEVIATION/MATLAB Function1 ==
  data: u1 input; y output
function y = fcn(u1)

y = ones(length(u1),1);

== matlab function TOGGLER/Subsystem4/Subsystem3/WFC Time Manager/ControlLogic_DEVIATION/MATLAB Function2 ==
  data: u1 input; u2 input; y output; u3 input
function y = fcn(u1, u2, u3)

if u3==0
    
    y = u2;
    return
end


u2(u3) = u1;

y = u2;

== matlab function TOGGLER/Subsystem4/Subsystem3/WFC Time Manager/ControlLogic_DEVIATION/MATLAB Function3 ==
  data: u1 input; y output; u2 input
function y = fcn(u1, u2)
if u2 == 0
    y = 0;
    return
end
    
    
y = u1(u2);

== matlab function TOGGLER/Subsystem4/MATLAB Function1 ==
  data: SectStrategies input; available output; CTRLList input
function available = fcn(SectStrategies, CTRLList)

available = zeros(length(CTRLList),1);
for iL = 1 : length(CTRLList)

 if sum(CTRLList(iL)==SectStrategies)
     available(iL,1) = 1;
 end
     
end

== matlab function TOGGLER/Subsystem4/MATLAB Function ==
  data: SectStrategies input; available output; CTRLList input
function available = fcn(SectStrategies, CTRLList)

available = zeros(length(CTRLList),1);
for iL = 1 : length(CTRLList)

 if sum(CTRLList(iL)==SectStrategies)
     available(iL,1) = 1;
 end
     
end

== matlab function TOGGLER/WDirCheck/Subsystem5/MATLAB Function ==
  data: u input; s output; N input
function s = fcn(u,N)

s = 0j;
for kk=1:N
    s = s + u(kk);
end

== matlab function TOGGLER/Subsystem4/Subsystem/Toggler ==
  data: AvailableCTRL input; CTRLList input; OldActiveCTRL input; ActiveCTRL output size=1; Counter output size=1; OldCounter input; TogglingSamples input
function [ActiveCTRL, Counter] = fcn(AvailableCTRL, CTRLList, OldActiveCTRL,  OldCounter, TogglingSamples)

idxOldActive = 0;
for iL = 1 : length(AvailableCTRL)
    if CTRLList(iL) == OldActiveCTRL
        idxOldActive = iL;
    end
end

    
% Analyze Available inputs

if OldActiveCTRL == 0 || sum(AvailableCTRL) == 0 %First Cycle or No control is active
    
    if sum(AvailableCTRL) == 0
        
        ActiveCTRL = 0;
    else
        
        TmpCTRLidx = 1;
        while ~AvailableCTRL(TmpCTRLidx)
            TmpCTRLidx = TmpCTRLidx + 1;
            if (TmpCTRLidx > length(AvailableCTRL))
                TmpCTRLidx = 1;
            end
        end
        ActiveCTRL = CTRLList(TmpCTRLidx);
        
    end
    
    Counter = 0;
    
else  % If another control is active, do the toggling


    
    TmpCTRLidx = mod(idxOldActive, length(AvailableCTRL)) + 1 ;
    while ~AvailableCTRL(TmpCTRLidx) 
        TmpCTRLidx = mod(TmpCTRLidx, length(AvailableCTRL)) + 1 ;
    end
    NextActiveCTRL = CTRLList(TmpCTRLidx);
    NextActiveIdx  = TmpCTRLidx;
    
    if  AvailableCTRL(idxOldActive) % Check time steps and change strategy if time is over
        
        if OldCounter < TogglingSamples
            Counter = OldCounter + 1;
            ActiveCTRL = OldActiveCTRL;
        else
            Counter = 0;
            ActiveCTRL = NextActiveCTRL;
            
        end
        
    else
        
        Counter = 0;
        ActiveCTRL = NextActiveCTRL;
        
    end
    
end


end

== matlab function TOGGLER/Subsystem4/Subsystem/WFC Time Manager/ControlLogic_DEVIATION/MATLAB Function ==
  data: CTRLToStopVec input; CTRLToSkip output; CTRLList input; iL output
function [CTRLToSkip, iL ] = fcn(CTRLToStopVec, CTRLList)

% y = u;
CTRLToSkip = 0;

for iL = 1 : length(CTRLList)
   if CTRLToStopVec(iL) > 0
     CTRLToSkip = CTRLList(iL);
     return
   end
    
end

if CTRLToSkip == 0
   iL =  0;
end

== matlab function TOGGLER/Subsystem4/Subsystem/WFC Time Manager/ControlLogic_DEVIATION/MATLAB Function1 ==
  data: u1 input; y output
function y = fcn(u1)

y = ones(length(u1),1);

== matlab function TOGGLER/Subsystem4/Subsystem/WFC Time Manager/ControlLogic_DEVIATION/MATLAB Function2 ==
  data: u1 input; u2 input; y output; u3 input
function y = fcn(u1, u2, u3)

if u3==0
    
    y = u2;
    return
end


u2(u3) = u1;

y = u2;

== matlab function TOGGLER/Subsystem4/Subsystem/WFC Time Manager/ControlLogic_DEVIATION/MATLAB Function3 ==
  data: u1 input; y output; u2 input
function y = fcn(u1, u2)
if u2 == 0
    y = 0;
    return
end
    
    
y = u1(u2);

== matlab function TOGGLER/Subsystem4/Subsystem3/Toggler ==
  data: AvailableCTRL input; CTRLList input; OldActiveCTRL input; ActiveCTRL output size=1; Counter output size=1; OldCounter input; TogglingSamples input
function [ActiveCTRL, Counter] = fcn(AvailableCTRL, CTRLList, OldActiveCTRL,  OldCounter, TogglingSamples)

% AvailableCTRL = logical([1 0 1])';
% CTRLList = [1 2 3]';
% OldActiveCTRL = 0;
% TogglingSamples = 2000;
% OldCounter = 0;


idxOldActive = 0;
for iL = 1 : length(AvailableCTRL)
    if CTRLList(iL) == OldActiveCTRL
        idxOldActive = iL;
    end
end

    
% Analyze Available inputs
% AvailableCTRLList = CTRLList(AvailableCTRL);

if OldActiveCTRL == 0 || sum(AvailableCTRL) == 0 %First Cycle or No control is active
    
    if sum(AvailableCTRL) == 0
        
        ActiveCTRL = 0;
    else
        
        TmpCTRLidx = 1;
        while ~AvailableCTRL(TmpCTRLidx)
            TmpCTRLidx = TmpCTRLidx + 1;
            if (TmpCTRLidx > length(AvailableCTRL))
                TmpCTRLidx = 1;
            end
        end
        ActiveCTRL = CTRLList(TmpCTRLidx);
        
    end
    
    Counter = 0;
    
else  % If another control is active, do the toggling


    
    TmpCTRLidx = mod(idxOldActive, length(AvailableCTRL)) + 1 ;
    while ~AvailableCTRL(TmpCTRLidx) 
        TmpCTRLidx = mod(TmpCTRLidx, length(AvailableCTRL)) + 1 ;
    end
    NextActiveCTRL = CTRLList(TmpCTRLidx);
    NextActiveIdx  = TmpCTRLidx;
    
    if  AvailableCTRL(idxOldActive) % Check time steps and change strategy if time is over
        
        if OldCounter < TogglingSamples
            Counter = OldCounter + 1;
            ActiveCTRL = OldActiveCTRL;
        else
            Counter = 0;
            ActiveCTRL = NextActiveCTRL;
            
        end
        
    else
        
        Counter = 0;
        ActiveCTRL = NextActiveCTRL;
        
    end
    
end


end

== matlab function TOGGLER/Subsystem4/Subsystem3/WFC Time Manager/ControlLogic_DEVIATION/MATLAB Function ==
  data: CTRLToStopVec input; CTRLToSkip output; CTRLList input; iL output
function [CTRLToSkip, iL ] = fcn(CTRLToStopVec, CTRLList)

% y = u;
CTRLToSkip = 0;

for iL = 1 : length(CTRLList)
   if CTRLToStopVec(iL) > 0
     CTRLToSkip = CTRLList(iL);
     return
   end
    
end

if CTRLToSkip == 0
   iL =  0;
end
